simulink model "threeservos"  (Simulink 4.00)
settings: Solver=ode45  StartTime=0.0  StopTime=1  RelTol=1e-3
InitFcn:
  | clear functions
libraries: truetime x1
settings Model: Creator=anton  LastModifiedBy=anton  LimitDataPoints=off  ExtModeTrigMode=oneshot  ExtModeArmWhenConnect=off  ExtModeAutoUpdateStatusClock=off  BlockReductionOpt=off

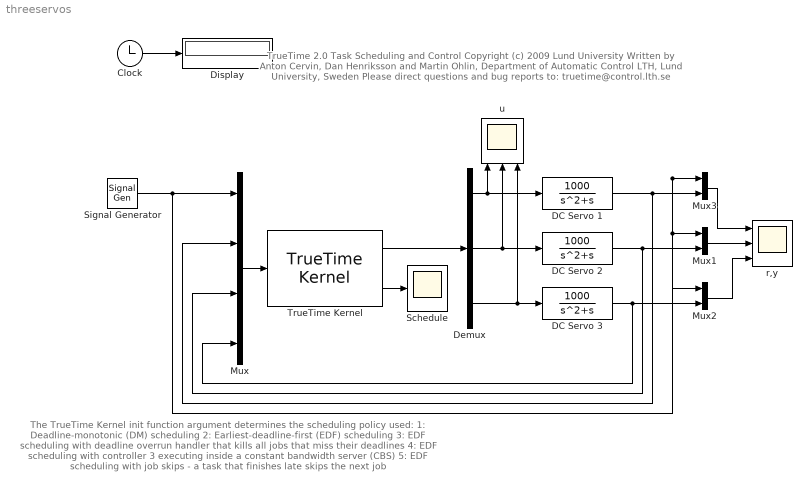
== system threeservos ==
  note: The TrueTime Kernel init function argument determines the scheduling policy used:
      |   1: Deadline-monotonic (DM) scheduling
      |   2: Earliest-deadline-first (EDF) scheduling
      |   3: EDF scheduling with deadline overrun handler that kills all jobs that miss their deadlines
      |   4: EDF scheduling with controller 3 executing inside a constant bandwidth server (CBS)
      |   5: EDF scheduling with job skips - a task that finishes late skips the next job
  note: TrueTime 2.0  Task Scheduling and Control
      | Copyright (c) 2009 Lund University
      | Written by Anton Cervin, Dan Henriksson and Martin Ohlin,
      | Department of Automatic Control LTH, Lund University, Sweden
      | Please direct questions and bug reports to:  truetime@control.lth.se
  Clock : Clock
      settings: DisplayTime=off  Decimation=10
  DC Servo 1 : TransferFcn  Numerator=[1000]  Denominator=[1 1 0]  AbsoluteTolerance=auto  Realization=auto
  DC Servo 2 : TransferFcn  Numerator=[1000]  Denominator=[1 1 0]  AbsoluteTolerance=auto  Realization=auto
  DC Servo 3 : TransferFcn  Numerator=[1000]  Denominator=[1 1 0]  AbsoluteTolerance=auto  Realization=auto
  Demux : Demux  Outputs=3  BusSelectionMode=off
  Display : Display
      settings: Format=short
  Mux : Mux  Inputs=4
  Mux1 : Mux  Inputs=2
  Mux2 : Mux  Inputs=2
  Mux3 : Mux  Inputs=2
  Schedule : Scope
      settings: TimeRange=1  YMin=1  YMax=3.5  SaveName=ry  MaxDataPoints=5000
  Signal Generator : SignalGenerator  WaveForm=square  Amplitude=1  Frequency=1.5  Units=Hertz
  TrueTime Kernel : truetime/TrueTime Kernel  sfun=threeservos_init  args=1  ninputsoutputs=[4 3]  ntriggers=0  trigtype=falling  nwnodenbr=[]  clockoffsetdrift=[0 0]  schedoutput=on  battery=off  poweroutput=off
  r,y : Scope  NumInputPorts=3
      settings: TimeRange=1  YMin=-2~-2~-2  YMax=2~2~2  SaveName=ry1  MaxDataPoints=5000
  u : Scope  NumInputPorts=3
      settings: Orientation=up  TimeRange=1  YMin=-2~-5~-5  YMax=2~5~5  SaveToWorkspace=off  SaveName=ScopeData  MaxDataPoints=5000
  wires:
  Clock/1 -> Display/1
  Signal Generator/1 -> Mux1/1, Mux2/1, Mux3/1, Mux/1
  Demux/2 -> DC Servo 2/1, u/2
  Demux/3 -> DC Servo 3/1, u/3
  DC Servo 1/1 -> Mux3/2, Mux/2
  DC Servo 2/1 -> Mux1/2, Mux/3
  DC Servo 3/1 -> Mux2/2, Mux/4
  Mux2/1 -> r,y/3
  Mux/1 -> TrueTime Kernel/1
  TrueTime Kernel/1 -> Demux/1
  Mux1/1 -> r,y/2
  Mux3/1 -> r,y/1
  Demux/1 -> DC Servo 1/1, u/1
  TrueTime Kernel/2 -> Schedule/1
